simulink model "motorai"  (R2018b)
settings: Solver=FixedStepAuto  StartTime=0.0  StopTime=inf  FixedStep=SAMPLE_TIME  RelTol=1e-3
PreLoadFcn:
  | UserSettings
InitFcn:
  | ESTIMATION_SAMPLES = 50;
values from neighbouring files (symbols this model uses):
  ADC_bits = 12    [LQR_control_design.m]    (also in UserSettings.m)
  ADC_Vref = 3.3    [LQR_control_design.m]    (also in UserSettings.m)
  current_gain = 0.5    [LQR_control_design.m]    (also in UserSettings.m)
  current_offset = 1    [LQR_control_design.m]    (also in UserSettings.m)
  DATA_SAMPLING_FREQUENCY = 500    [UserSettings.m]
  K = -K    (= -0.383)    [LQG_control_design.m]    (also in LQR_control_design.m = -(1/R).*B'*Sinf; myLQR.m = -(1/R).*B'*Sinf; myREF.m = [Kw Ki])
  motorParameters = Parameters()    [UserSettings.m]
  omega_gain = 0.5    [LQR_control_design.m]    (also in UserSettings.m)
  omega_offset = 1    [LQR_control_design.m]    (also in UserSettings.m)
  PPR = 1000    [LQR_control_design.m]    (also in UserSettings.m)
  Q = 1/2*inv([(omega_max)^2 0 0; 0 (i_max)^2 0; 0 0 (int_max)^2])    [LQG_control_design.m]    (also in LQR_control_design.m = 1/2*inv([(omega_max)^2 0 ; 0 (i_max)^2]); myLQR.m = 1/2*inv([(omega_max)^2 0; 0 (i_max)^2]))
  R = inv([(v_max)^2])    [LQG_control_design.m]    (also in LQR_control_design.m; myLQR.m)
  SAMPLE_TIME = 5e-5    (= 5e-05)    [UserSettings.m]
  V_ACT = 12    [UserSettings.m]
  Vact = 12    [LQR_control_design.m]
undefined symbols (not defined in the file or in its folder): DiscIntNeverNeededParam
libraries: neural x275, mbedblockslib x7, fl_lib x5, nesl_utility x5, dspswit3 x3, elec_lib x3, powerlib_meascontrol x3, dspbuff3 x2, discretizing x1
(part 14 of 14)

== system motorai/Parameter Estimation & LQR /Function Fitting Neural Network1/Layer 3/Delays 1 ==
  "p{3}" : Inport  PortDimensions=54
      mask Display: e = 0.06;c1 = [120 230 180]/255;c2 = ([120 230 180]+0)/(256+128);c3 = ([120 230 180]+128)/(256+128);patch([0 1 1 0],[0 0 1 1],c1);patch([0 1 1 1-e 1-e 0+e],[0 0 1 1-e 0+e 0+e],c2);patch([0 0 1 1-e 0+e 0+e],[0 1 1 1-e 1-e 0+e],c3);plot([0 1 1 0 0],[0 0 1 1 0]);
  mux : Mux  Inputs=1
      mask Display: e = 0.06;c1 = [120 150 230]/255;c2 = ([120 150 230]+0)/383;c3 = ([120 150 230]+128)/383;patch([0 1 1 0],[0 0 1 1],c1);patch([0 1 1 1-e 1-e 0+e],[0 0 1 1-e 0+e 0+e],c2);patch([0 0 1 1-e 0+e 0+e],[0 1 1 1-e 1-e 0+e],c3);plot([0 1 1 0 0],[0 0 1 1 0]);disp('Mux')
  "pd{3,2}" : Outport
      mask Display: e = 0.06;c1 = [120 230 180]/255;c2 = ([120 230 180]+0)/(256+128);c3 = ([120 230 180]+128)/(256+128);patch([0 1 1 0],[0 0 1 1],c1);patch([0 1 1 1-e 1-e 0+e],[0 0 1 1-e 0+e 0+e],c2);patch([0 0 1 1-e 0+e 0+e],[0 1 1 1-e 1-e 0+e],c3);plot([0 1 1 0 0],[0 0 1 1 0]);
  wires:
  "p{3}"/1 -> mux/1
  mux/1 -> "pd{3,2}"/1

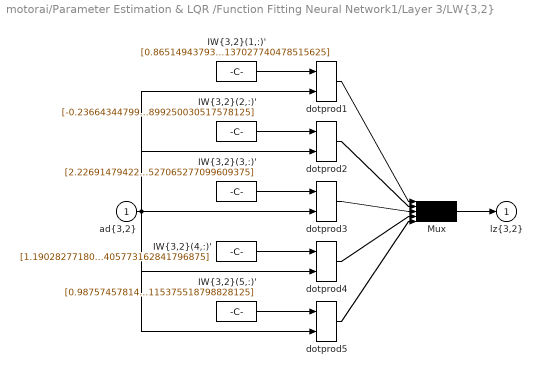
== system motorai/Parameter Estimation & LQR /Function Fitting Neural Network1/Layer 3/LW{3,2} ==
  "ad{3,2}" : Inport  PortDimensions=54
      mask Display: e = 0.06;c1 = [120 230 180]/255;c2 = ([120 230 180]+0)/(256+128);c3 = ([120 230 180]+128)/(256+128);patch([0 1 1 0],[0 0 1 1],c1);patch([0 1 1 1-e 1-e 0+e],[0 0 1 1-e 0+e 0+e],c2);patch([0 0 1 1-e 0+e 0+e],[0 1 1 1-e 1-e 0+e],c3);plot([0 1 1 0 0],[0 0 1 1 0]);
  "IW{3,2}(1,:)'" : Constant  Value=[0.86514943793769838453755482987617142498493194580078125;1.0695933378726707463357570304651744663715362548828125;-0.5712362276227909152481743149110116064548492431640625;0.228026730829081258900004058887134306132793426513671875;2.971384076008977803695643160608597099781036376953125;-2.457674822110419654563884250819683074951171875;-0.98379412060172499732146889073192141950130462646484375;0.233434941324575095933369084377773106098175048828125;-0.312324929667214867823332724583451636135578155517578125;-0.377019122929658667686680928454734385013580322265625;0.0301808166691558132921358037492609582841396331787109375;-0.489331002697269312751160441621323116123676300048828125;-0.21676323897270022289518465186120010912418365478515625;1.036218083155919345017537125386297702789306640625;0.34267571081690129108920928047155030071735382080078125;1.3932949674386361227362840509158559143543243408203125;-0.42499274383423524259484338472248055040836334228515625;1.117876766730884430245396288228221237659454345703125;0.57649388577341242889673367244540713727474212646484375;0.2423141368071626278180019653518684208393096923828125;-0.381851676403098416745507392988656647503376007080078125;-0.35382391063296536604099173928261734545230865478515625;0.27569673594311361330966292371158488094806671142578125;0.2048838230976395002880252604882116429507732391357421875;-0.3957117999871695435132323837024159729480743408203125;1.5264299108269392402092989868833683431148529052734375;1.61231862573349449263560018152929842472076416015625;-1.2386255874347458227902052385616116225719451904296875;1.1299053529005622653613727379706688225269317626953125;1.08968731861545808925484379869885742664337158203125;1.2305699078123149003971548154368065297603607177734375;0.73635826965319373105245404076413251459598541259765625;-0.357142162932608753234120513297966681420803070068359375;-0.3386881752262149714027827940299175679683685302734375;-0.1404648943518874981695176984430872835218906402587890625;0.95536711486602943210755256586708128452301025390625;-0.353425844518761966828179765798267908394336700439453125;-1.1083892529320660269576137579861097037792205810546875;-0.7833974136848953495615432984777726233005523681640625;-1.081846102399868669863280956633388996124267578125;-0.188907087493226655272593461631913669407367706298828125;0.1861017690661447565592112596277729608118534088134765625;0.53624445012368304741556812587077729403972625732421875;0.51217597170973672149330013780854642391204833984375;-0.470065529079076116492075243513681925833225250244140625;0.37662231402563062232502488768659532070159912109375;-0.254185698997341003035899120732210576534271240234375;0.396143697121934368343687538072117604315280914306640625;-2.287411364297277760471160945598967373371124267578125;-1.1542484397201044910019618328078649938106536865234375;-0.690170626866897674034362353268079459667205810546875;0.693129862216120162798915771418251097202301025390625;-0.40691380322596593099859774156357161700725555419921875;0.2826327304047409061382722939015366137027740478515625]
      mask Display: e = 0.06;c1 = [120 150 230]/255;c2 = ([120 150 230]+0)/383;c3 = ([120 150 230]+128)/383;patch([0 1 1 0],[0 0 1 1],c1);patch([0 1 1 1-e 1-e 0+e],[0 0 1 1-e 0+e 0+e],c2);patch([0 0 1 1-e 0+e 0+e],[0 1 1 1-e 1-e 0+e],c3);plot([0 1 1 0 0],[0 0 1 1 0]);disp('weights');
  "IW{3,2}(2,:)'" : Constant  Value=[-0.2366434479986641026272309318301267921924591064453125;-0.3981802925660435921173530005034990608692169189453125;0.224450636092790423159470947211957536637783050537109375;-0.386069362490764955708755223895423114299774169921875;-1.202091119457073364884536204044707119464874267578125;0.454347794383640646298516685419599525630474090576171875;1.3735952757409481961303754360415041446685791015625;0.461518611103885756374864968165638856589794158935546875;-1.436072129176569678321584433433599770069122314453125;-1.6789060123597454587951460780459456145763397216796875;1.8853755636739990553252255267580039799213409423828125;-0.141162648621668995740918717274325899779796600341796875;-0.2018905255054873337794418830526410602033138275146484375;0.84140936101645558142791969657992012798786163330078125;-0.9317143508376128924197701053344644606113433837890625;-3.214245195871603844040009789750911295413970947265625;-0.126861871578991924902624077731161378324031829833984375;0.17547455943169232295275605792994610965251922607421875;-0.84229212479691317749797008218592964112758636474609375;-0.1407913556871722426944160133643890731036663055419921875;-0.790907719324559277396247125579975545406341552734375;1.481518186897975652982495375908911228179931640625;0.320470972429969969130780782506917603313922882080078125;0.1921266655036854842375504404117236845195293426513671875;-1.0511433479165142035327562552993185818195343017578125;-2.752584848581496768105125738657079637050628662109375;-0.44127320826636651229790686556953005492687225341796875;2.869535429426183892331891911453567445278167724609375;0.1446204169352660329206372580301831476390361785888671875;-0.2185821943262183097989037605657358653843402862548828125;-0.275756850162166333717550514847971498966217041015625;0.174698574578167009629936501369229517877101898193359375;-1.1808792085189072640361018784460611641407012939453125;0.443946974458954646269859267704305239021778106689453125;-1.02214659651594086398063154774717986583709716796875;0.3363769758631367512435872413334436714649200439453125;-0.317155630204158656137991556533961556851863861083984375;-0.163015254128853925852382644734461791813373565673828125;0.86786367702748845598392790634534321725368499755859375;0.72311394086383484758329132091603241860866546630859375;3.267243281802581389428041802602820098400115966796875;-0.0177210428410714791735980355724677792750298976898193359375;-3.75571146579581949254134087823331356048583984375;-3.4523677230253699832474012509919703006744384765625;-0.75490473563561433234525566149386577308177947998046875;-2.0056063012150193713978296727873384952545166015625;0.98525944915435303972373048964072950184345245361328125;-0.342941673848266848079191504439222626388072967529296875;0.851777021508766996049644149024970829486846923828125;2.035716895915056223742567453882656991481781005859375;-1.2101614031539777993629058983060531318187713623046875;0.81647443962144528040170143867726437747478485107421875;0.264585765353807733646362976287491619586944580078125;-0.3202656238302445945720364761655218899250030517578125]
      mask Display: e = 0.06;c1 = [120 150 230]/255;c2 = ([120 150 230]+0)/383;c3 = ([120 150 230]+128)/383;patch([0 1 1 0],[0 0 1 1],c1);patch([0 1 1 1-e 1-e 0+e],[0 0 1 1-e 0+e 0+e],c2);patch([0 0 1 1-e 0+e 0+e],[0 1 1 1-e 1-e 0+e],c3);plot([0 1 1 0 0],[0 0 1 1 0]);disp('weights');
  "IW{3,2}(3,:)'" : Constant  Value=[2.2269147942210310020527685992419719696044921875;-0.247338650477427923757289818240678869187831878662109375;1.0058555297725420007992624960024841129779815673828125;-0.33323080042560648816873936084448359906673431396484375;-0.96353933335864250242508433075272478163242340087890625;4.61669793309417375581915621296502649784088134765625;1.1497034258122038608007642324082553386688232421875;-0.0325848597359635061554428148156148381531238555908203125;-0.356807752024108137955948905073455534875392913818359375;-1.3218225961301761639532514891470782458782196044921875;1.7568830951932541406534937777905724942684173583984375;0.87020944697544333479299893951974809169769287109375;-0.0983143960217268408907642651684000156819820404052734375;-0.387165659394644146029662579167052172124385833740234375;-1.016126961942592554777320401626639068126678466796875;0.56039479141408443663152638691826723515987396240234375;0.05462371745566728387100141617338522337377071380615234375;-0.125283905375902282486322292243130505084991455078125;0.7027262142897734431556955314590595662593841552734375;-2.11256743084311349178960881545208394527435302734375;-0.2213453504696782647709341063091414980590343475341796875;0.1512422890359938210114165713093825615942478179931640625;-0.35462120149324583007199862549896351993083953857421875;-0.2191358086332166610343819002082454971969127655029296875;-0.324901619311246447896479594419361092150211334228515625;1.4520792571257963299302673476631753146648406982421875;-0.025598804118970135135224808209386537782847881317138671875;-0.5919979018295677963834577894886024296283721923828125;-1.936431630432263073515741780283860862255096435546875;-0.9302664122991470829759919070056639611721038818359375;1.4448187703593828867809634175500832498073577880859375;0.487698303949225142606138660994474776089191436767578125;-0.397395398451121539817876282540964893996715545654296875;0.9624250930564237638265012719784863293170928955078125;-0.06923450739827341493537460337392985820770263671875;1.039626267968295270094358784263022243976593017578125;1.9302642873497861675247122548171319067478179931640625;-0.07352757545522148330263689786079339683055877685546875;1.06326186660250954219009145162999629974365234375;-1.2510041543824959031638854867196641862392425537109375;0.3157979558899481897782379746786318719387054443359375;-0.2388620487784617052451352492425939999520778656005859375;-0.353399007038871004748870063849608413875102996826171875;-0.39418719724949458083074205205775797367095947265625;-0.488980033653386048086986193084158003330230712890625;-1.4034826322450992819312887149862945079803466796875;-1.4234402809959798563710364760481752455234527587890625;0.748576394444523174342975835315883159637451171875;0.70529374566448488348413548010285012423992156982421875;0.853852099750808779532462722272612154483795166015625;-0.17956164085841475053229032710078172385692596435546875;0.64782968689951492269329946793732233345508575439453125;-0.433809209903048331735675446907407604157924652099609375;2.276931715932169364435821989900432527065277099609375]
      mask Display: e = 0.06;c1 = [120 150 230]/255;c2 = ([120 150 230]+0)/383;c3 = ([120 150 230]+128)/383;patch([0 1 1 0],[0 0 1 1],c1);patch([0 1 1 1-e 1-e 0+e],[0 0 1 1-e 0+e 0+e],c2);patch([0 0 1 1-e 0+e 0+e],[0 1 1 1-e 1-e 0+e],c3);plot([0 1 1 0 0],[0 0 1 1 0]);disp('weights');
  "IW{3,2}(4,:)'" : Constant  Value=[1.1902827718005486445917995297349989414215087890625;0.567072384614290658788604559958912432193756103515625;-0.186810501416461660628698382424772717058658599853515625;-0.5047614479402369180860432607005350291728973388671875;0.0031542921314069252182454849986470435396768152713775634765625;3.057037170730933173246057776850648224353790283203125;-1.137952949114983791645272503956221044063568115234375;-2.4303779842662240895378999994136393070220947265625;-0.7695152047852771293179330314160324633121490478515625;0.644492590531159148525830460130237042903900146484375;-0.351806183792259641318622698236140422523021697998046875;-0.83784820783761515539111996986321173608303070068359375;-0.016999433581893062805701077877529314719140529632568359375;-1.2300467578103579935344669138430617749691009521484375;-0.94649445563016509908038642606697976589202880859375;0.59540623082449106728830656720674596726894378662109375;-1.76291183936469497695043173735029995441436767578125;0.630195682219659492062646677368320524692535400390625;1.2939119923943465106930261754314415156841278076171875;0.5890207720839255589595495621324516832828521728515625;1.547368313650863580477334835450164973735809326171875;0.294767781513982696228737268029362894594669342041015625;-1.7747129253234390500182371397386305034160614013671875;-2.909300845333242957480024415417574346065521240234375;0.9351344326501489501168862261692993342876434326171875;-0.85019601787469145648401536163873970508575439453125;0.82614647447679756542271434227586723864078521728515625;-0.62168238952753041015597545992932282388210296630859375;-2.100571483518670401480221698875539004802703857421875;6.75874068219558044035011334926821291446685791015625;-0.53899026172956709945793818405945785343647003173828125;-0.541114414429402668105240081786178052425384521484375;0.5082597602030272110340547442319802939891815185546875;-0.90220742578864843164154763144324533641338348388671875;0.08729926326432059513482641932569094933569431304931640625;0.255927081232561193235852670113672502338886260986328125;-2.849833054174956803450413644895888864994049072265625;0.55885597208317339124050704413093626499176025390625;-3.221788949249335676228156444267369806766510009765625;-0.71551893204270700099556279383250512182712554931640625;0.14976350889207956651461017827386967837810516357421875;-0.694416698267585896786613375297747552394866943359375;-0.8269744567607391072527889264165423810482025146484375;-0.217518949230630365132554970841738395392894744873046875;1.39973408639140739495587695273570716381072998046875;2.164776195210448950234649601043201982975006103515625;-2.18349724034951098161627669469453394412994384765625;-1.3764526359715423264873379594064317643642425537109375;0.0686248541682902002403210417469381354749202728271484375;-1.68664782072590213601870345883071422576904296875;0.34968792815968707810014848291757516562938690185546875;1.6227683012909988047312026537838391959667205810546875;-0.003693971508892235529331049548318333108909428119659423828125;0.63667810145512060415740052121691405773162841796875]
      mask Display: e = 0.06;c1 = [120 150 230]/255;c2 = ([120 150 230]+0)/383;c3 = ([120 150 230]+128)/383;patch([0 1 1 0],[0 0 1 1],c1);patch([0 1 1 1-e 1-e 0+e],[0 0 1 1-e 0+e 0+e],c2);patch([0 0 1 1-e 0+e 0+e],[0 1 1 1-e 1-e 0+e],c3);plot([0 1 1 0 0],[0 0 1 1 0]);disp('weights');
  "IW{3,2}(5,:)'" : Constant  Value=[0.98757457814580751342958819805062375962734222412109375;0.03184348396875412434692265151170431636273860931396484375;0.1001380751692779735861904555349610745906829833984375;-0.24731743099228686855184378146077506244182586669921875;-3.531547045912895921304652802064083516597747802734375;-2.332740840955342065399236162193119525909423828125;0.340480871157649300773329059666139073669910430908203125;0.323864539557960184890106347666005603969097137451171875;0.63170752218164694102853218282689340412616729736328125;-0.2816846762684657168307467145496048033237457275390625;-0.10039198525839047870800158079873654060065746307373046875;0.1370292589029349084039921535804751329123973846435546875;0.66752839301872024524442394977086223661899566650390625;-0.61363427884571819515002744083176366984844207763671875;0.65412230667584136956094198467326350510120391845703125;0.3302764738029513313932739038136787712574005126953125;-0.59493462992305656822367154745734296739101409912109375;-0.4947862965777307664438922074623405933380126953125;-1.822514713166993427506668012938462197780609130859375;-1.2806700886065549571668498174403794109821319580078125;-0.5742144707313323603870003353222273290157318115234375;-0.208295132246331837766462058425531722605228424072265625;-0.296384462947958449152707771645509637892246246337890625;-0.452998404504511731349936098922626115381717681884765625;0.67305461656774079326481796670123003423213958740234375;0.48519511227910017137077147708623670041561126708984375;-0.61214368567271104648597201958182267844676971435546875;-0.3491749935402810312012888971366919577121734619140625;2.483367685024400639548503022524528205394744873046875;-0.32371639439706212382219518985948525369167327880859375;1.3249208873568092403871787610114552080631256103515625;0.85823606136657393239630664538708515465259552001953125;-0.62058104329758700945518512526177801191806793212890625;0.44108797716339054328926749803940765559673309326171875;-1.049379221026043751407996751368045806884765625;0.0042613459464942715637647552284761331975460052490234375;2.60290659793950052147692986181937158107757568359375;0.7068172103118757210182820927002467215061187744140625;0.54053366532072166794620216023758985102176666259765625;-0.75757064498732074042663953150622546672821044921875;-0.396128164223576495484024917459464631974697113037109375;-0.00230329664144797961744526304528335458599030971527099609375;-0.0133866411608924186504854247914408915676176548004150390625;0.4045282880433040961776214317069388926029205322265625;-0.164073618594850423324515986678306944668292999267578125;-1.3319462771611341178612519797752611339092254638671875;-1.2150359807785851007366773046669550240039825439453125;-0.69232271647843479644990338783827610313892364501953125;3.228561441752543004213293897919356822967529296875;-0.54051597431018627570864509834791533648967742919921875;0.40743457955528772362896461345371790230274200439453125;-0.012379078876847936230287672287886380217969417572021484375;0.2036410621633234219185482061220682226121425628662109375;1.5840991985147514498066811938770115375518798828125]
      mask Display: e = 0.06;c1 = [120 150 230]/255;c2 = ([120 150 230]+0)/383;c3 = ([120 150 230]+128)/383;patch([0 1 1 0],[0 0 1 1],c1);patch([0 1 1 1-e 1-e 0+e],[0 0 1 1-e 0+e 0+e],c2);patch([0 0 1 1-e 0+e 0+e],[0 1 1 1-e 1-e 0+e],c3);plot([0 1 1 0 0],[0 0 1 1 0]);disp('weights');
  Mux : Mux  Inputs=5
      mask Display: e = 0.06;c1 = [120 150 230]/255;c2 = ([120 150 230]+0)/383;c3 = ([120 150 230]+128)/383;patch([0 1 1 0],[0 0 1 1],c1);patch([0 1 1 1-e 1-e 0+e],[0 0 1 1-e 0+e 0+e],c2);patch([0 0 1 1-e 0+e 0+e],[0 1 1 1-e 1-e 0+e],c3);plot([0 1 1 0 0],[0 0 1 1 0]);disp('Mux');
  dotprod{1..5} (5 alike) : neural/Weight Functions/dotprod
  "lz{3,2}" : Outport
      mask Display: e = 0.06;c1 = [120 230 180]/255;c2 = ([120 230 180]+0)/(256+128);c3 = ([120 230 180]+128)/(256+128);patch([0 1 1 0],[0 0 1 1],c1);patch([0 1 1 1-e 1-e 0+e],[0 0 1 1-e 0+e 0+e],c2);patch([0 0 1 1-e 0+e 0+e],[0 1 1 1-e 1-e 0+e],c3);plot([0 1 1 0 0],[0 0 1 1 0]);
  wires:
  "IW{3,2}(1,:)'"/1 -> dotprod1/1
  "ad{3,2}"/1 -> dotprod1/2, dotprod2/2, dotprod3/2, dotprod4/2, dotprod5/2
  dotprod1/1 -> Mux/1
  "IW{3,2}(2,:)'"/1 -> dotprod2/1
  dotprod2/1 -> Mux/2
  "IW{3,2}(3,:)'"/1 -> dotprod3/1
  dotprod3/1 -> Mux/3
  "IW{3,2}(4,:)'"/1 -> dotprod4/1
  dotprod4/1 -> Mux/4
  "IW{3,2}(5,:)'"/1 -> dotprod5/1
  dotprod5/1 -> Mux/5
  Mux/1 -> "lz{3,2}"/1

== stateflow chart motorai/Logic Brain1 ==
  state idle
    entry:
    start_signal = 0;
  state start_estimation
    entry:
    start_signal = 1;
    during:
    start_signal = 1;
  (default) -> idle
  idle -> start_estimation : [button == 1]
  start_estimation -> idle : [stop_signal==1]
  data: stop_signal input; start_button input; start_signal output

== stateflow chart motorai/Logic Brain ==
  state idle
    entry:
    start_signal = 0;
  state start_estimation
    entry:
    start_signal = 1;
  state button_wait
  (default) -> idle
  start_estimation -> idle : [stop_signal > 0]{reset = 1}
  idle -> button_wait : [start_button == 1]{n_stop_motor = 0}
  button_wait -> start_estimation [order 2] : [start_button == 0]{reset = 0, n_stop_motor = 1}
  button_wait -> button_wait [order 1] : [start_button == 1]
  data: stop_signal input; start_button input; reset output; start_signal output =0; n_stop_motor output

== matlab function motorai/Parameter Estimation & LQR /MATLAB Function ==
  data: R input; A output; L input; Km input; Bm input; I input; B output; C output
function [A,B,C] = SystemMatrices(R, L, Km, Bm, I)
%---System Matrices----------------------------------------------
%---| x = Ax + Bu |----------------------------------------------
%---| y = Cx      |----------------------------------------------
A = [-Bm/I Km/I; -Km/L -R/L];
B = [0; 1/L];
C = [1 0];

== matlab function motorai/Parameter Estimation & LQR /MATLAB Function1 ==
  data: A input; K output; B input; Q input; R input
function K = myLQR(A,B,Q,R)

%RICCATI  Solves an algebraic Riccati equation
%   X = Riccati(A,G,Q) solves the algebraic Riccati equation of the form:
%       A'*X + X*A' - X*G*X + Q = 0, where X is symmetric.
   n=size(A,1);
   G = zeroes(n);
   H = zeroes(2*n);

   G = (1/R).*B*B';

   H = [A -G
       -Q -A'];

   [U,~] = schur(H);
   %[U,S]=ordschur(U1,S1,'lhp');

   X = U(n+1:end,1:n)*U(1:n,1:n)^-1;
%end RICCATI

Sinf = X;
   
K = -(1/R).*B'*Sinf;
